simulink model "rigid_6dof"  (R2017a)
settings: Solver=FixedStepAuto  StartTime=0.0  StopTime=sim_duration  FixedStep=sim_step  RelTol=1e-3
libraries: shared6dof x1
settings Model: Creator=root  LastModifiedBy=root
settings DataIOCC: SaveOutput=off  SignalLogging=off  DSMLogging=off  SaveTime=off

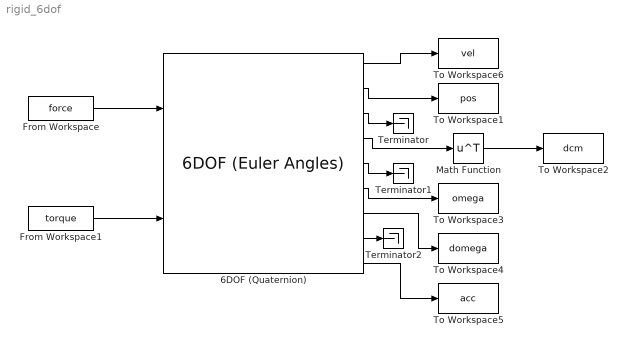
== system rigid_6dof ==
  6DOF (Quaternion) : shared6dof/6DOF (Euler Angles)  units=Metric (MKS)  mtype=Fixed  rep=Quaternion  xme_0=pos_0  Vm_0=vel_0  eul_0=euler_0  pm_0=omega_0  mass_0=1.0  mass_e=0.5  mass_f=2.0  inertia=eye(3)  inertia_e=eye(3)  inertia_f=2*eye(3)  k_quat=1.0  vre_flag=on  abi_flag=on
      settings: SourceProductName=Attempt to write the readonly database /home/mr/.matlab/R2017a/slblocks_master.db. (attempt to write a readonly database)
  From Workspace : FromWorkspace  VariableName=force  SampleTime=0
  From Workspace1 : FromWorkspace  VariableName=torque  SampleTime=0
  Math Function : Math  Operator=transpose  SaturateOnIntegerOverflow=on
  Terminator : Terminator
  Terminator1 : Terminator
  Terminator2 : Terminator
  To Workspace1 : ToWorkspace  VariableName=pos  SaveFormat=Timeseries  SampleTime=-1
  To Workspace2 : ToWorkspace  VariableName=dcm  SaveFormat=Timeseries  SampleTime=-1
  To Workspace3 : ToWorkspace  VariableName=omega  SaveFormat=Timeseries  SampleTime=-1
  To Workspace4 : ToWorkspace  VariableName=domega  SaveFormat=Timeseries  SampleTime=-1
  To Workspace5 : ToWorkspace  VariableName=acc  SaveFormat=Timeseries  SampleTime=-1
  To Workspace6 : ToWorkspace  VariableName=vel  SaveFormat=Timeseries  SampleTime=-1
  wires:
  6DOF (Quaternion)/2 -> To Workspace1/1
  6DOF (Quaternion)/6 -> To Workspace3/1
  6DOF (Quaternion)/7 -> To Workspace4/1
  6DOF (Quaternion)/9 -> To Workspace5/1
  6DOF (Quaternion)/3 -> Terminator/1
  6DOF (Quaternion)/5 -> Terminator1/1
  From Workspace/1 -> 6DOF (Quaternion)/1
  From Workspace1/1 -> 6DOF (Quaternion)/2
  6DOF (Quaternion)/1 -> To Workspace6/1
  6DOF (Quaternion)/8 -> Terminator2/1
  6DOF (Quaternion)/4 -> Math Function/1
  Math Function/1 -> To Workspace2/1
